simulink model "fxpdemo_sfun_user_U32BitRegion"  (Simulink 7.6)
settings: Solver=FixedStepDiscrete  StartTime=0.0  StopTime=1  FixedStep=0.001  RelTol=1e-3
libraries: simulink x8
settings Model: Creator=The MathWorks Inc.  ExtModeAutoUpdateStatusClock=off
settings OptimizationCC: InitFltsAndDblsToZero=on
settings DebuggingCC: StrictBusMsg=Warning

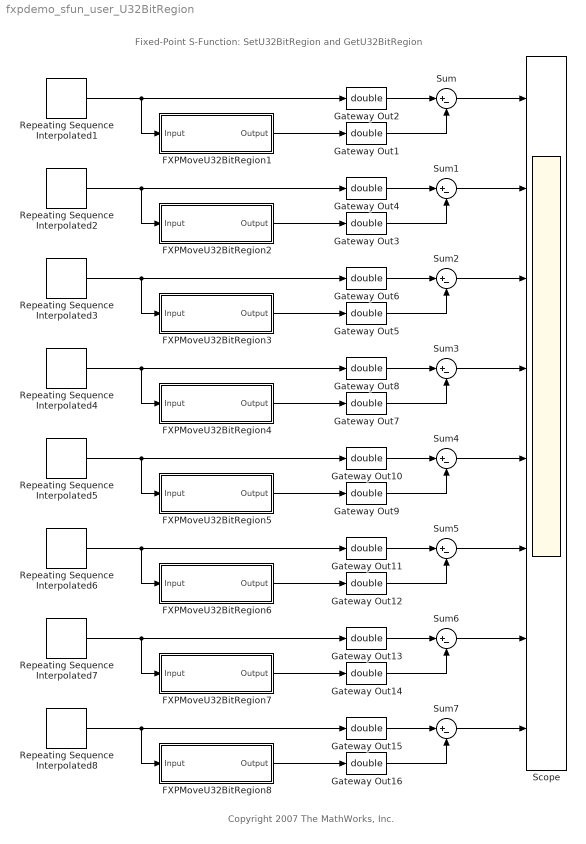
== system fxpdemo_sfun_user_U32BitRegion ==
  note: Fixed-Point S-Function: SetU32BitRegion and GetU32BitRegion
  note: Copyright 2007 The MathWorks, Inc.
  FXPMoveU32BitRegion1 : Subsystem
  FXPMoveU32BitRegion2 : Subsystem
  FXPMoveU32BitRegion3 : Subsystem
  FXPMoveU32BitRegion4 : Subsystem
  FXPMoveU32BitRegion5 : Subsystem
  FXPMoveU32BitRegion6 : Subsystem
  FXPMoveU32BitRegion7 : Subsystem
  FXPMoveU32BitRegion8 : Subsystem
  Gateway Out{1..16} (16 alike) : DataTypeConversion  OutDataTypeStr=double  RndMeth=Zero
  Repeating Sequence Interpolated1 : simulink/Sources/Repeating Sequence Interpolated  SystemSampleTime=-1  OutValues=0+2*[0 0.25 0.5 0.75 1].'  TimeValues=[0 0.25 0.5 0.75 1].'  LookUpMeth=Interpolation-Use End Values  tsamp=0.001  OutMin=[]  OutMax=[]  OutDataTypeStr=fixdt(0,9,4)  OutputDataTypeScalingMode=Specify via dialog  OutDataType=ufix(9)  OutScaling=2^-4
  Repeating Sequence Interpolated2 : simulink/Sources/Repeating Sequence Interpolated  SystemSampleTime=-1  OutValues=0+2*[0 0.25 0.5 0.75 1].'  TimeValues=[0 0.25 0.5 0.75 1].'  LookUpMeth=Interpolation-Use End Values  tsamp=0.001  OutMin=[]  OutMax=[]  OutDataTypeStr=fixdt(0,17,6)  OutputDataTypeScalingMode=Specify via dialog  OutDataType=ufix(17)  OutScaling=2^-6
  Repeating Sequence Interpolated3 : simulink/Sources/Repeating Sequence Interpolated  SystemSampleTime=-1  OutValues=0+2*[0 0.25 0.5 0.75 1].'  TimeValues=[0 0.25 0.5 0.75 1].'  LookUpMeth=Interpolation-Use End Values  tsamp=0.001  OutMin=[]  OutMax=[]  OutDataTypeStr=fixdt(0,33,8)  OutputDataTypeScalingMode=Specify via dialog  OutDataType=ufix(33)  OutScaling=2^-8
  Repeating Sequence Interpolated4 : simulink/Sources/Repeating Sequence Interpolated  SystemSampleTime=-1  OutValues=0+2*[0 0.25 0.5 0.75 1].'  TimeValues=[0 0.25 0.5 0.75 1].'  LookUpMeth=Interpolation-Use End Values  tsamp=0.001  OutMin=[]  OutMax=[]  OutDataTypeStr=fixdt(0,65,10)  OutputDataTypeScalingMode=Specify via dialog  OutDataType=ufix(65)  OutScaling=2^-10
  Repeating Sequence Interpolated5 : simulink/Sources/Repeating Sequence Interpolated  SystemSampleTime=-1  OutValues=0+2*[0 0.25 0.5 0.75 1].'  TimeValues=[0 0.25 0.5 0.75 1].'  LookUpMeth=Interpolation-Use End Values  tsamp=0.001  OutMin=[]  OutMax=[]  OutDataTypeStr=fixdt(1,15,3)  OutputDataTypeScalingMode=Specify via dialog  OutDataType=sfix(15)  OutScaling=2^-3
  Repeating Sequence Interpolated6 : simulink/Sources/Repeating Sequence Interpolated  SystemSampleTime=-1  OutValues=0+2*[0 0.25 0.5 0.75 1].'  TimeValues=[0 0.25 0.5 0.75 1].'  LookUpMeth=Interpolation-Use End Values  tsamp=0.001  OutMin=[]  OutMax=[]  OutDataTypeStr=fixdt(1,31,6)  OutputDataTypeScalingMode=Specify via dialog  OutDataType=sfix(31)  OutScaling=2^-6
  Repeating Sequence Interpolated7 : simulink/Sources/Repeating Sequence Interpolated  SystemSampleTime=-1  OutValues=0+2*[0 0.25 0.5 0.75 1].'  TimeValues=[0 0.25 0.5 0.75 1].'  LookUpMeth=Interpolation-Use End Values  tsamp=0.001  OutMin=[]  OutMax=[]  OutDataTypeStr=fixdt(1,63,9)  OutputDataTypeScalingMode=Specify via dialog  OutDataType=sfix(63)  OutScaling=2^-9
  Repeating Sequence Interpolated8 : simulink/Sources/Repeating Sequence Interpolated  SystemSampleTime=-1  OutValues=0+2*[0 0.25 0.5 0.75 1].'  TimeValues=[0 0.25 0.5 0.75 1].'  LookUpMeth=Interpolation-Use End Values  tsamp=0.001  OutMin=[]  OutMax=[]  OutDataTypeStr=fixdt(1,127,12)  OutputDataTypeScalingMode=Specify via dialog  OutDataType=sfix(127)  OutScaling=2^-12
  Scope : Scope  NumInputPorts=8
      settings: YMin=-5~-5~-5~-5~-5~-5~-5~-5  YMax=5~5~5~5~5~5~5~5
  Sum{,1..7} (8 alike) : Sum  Inputs=|+-
  wires:
  Repeating Sequence Interpolated1/1 -> Gateway Out2/1, FXPMoveU32BitRegion1/1(Input)
  FXPMoveU32BitRegion1/1(Output) -> Gateway Out1/1
  Gateway Out2/1 -> Sum/1
  Gateway Out1/1 -> Sum/2
  Repeating Sequence Interpolated2/1 -> FXPMoveU32BitRegion2/1(Input), Gateway Out4/1
  FXPMoveU32BitRegion2/1(Output) -> Gateway Out3/1
  Gateway Out4/1 -> Sum1/1
  Gateway Out3/1 -> Sum1/2
  Repeating Sequence Interpolated3/1 -> Gateway Out6/1, FXPMoveU32BitRegion3/1(Input)
  FXPMoveU32BitRegion3/1(Output) -> Gateway Out5/1
  Gateway Out6/1 -> Sum2/1
  Gateway Out5/1 -> Sum2/2
  Repeating Sequence Interpolated4/1 -> FXPMoveU32BitRegion4/1(Input), Gateway Out8/1
  FXPMoveU32BitRegion4/1(Output) -> Gateway Out7/1
  Gateway Out8/1 -> Sum3/1
  Gateway Out7/1 -> Sum3/2
  Repeating Sequence Interpolated5/1 -> Gateway Out10/1, FXPMoveU32BitRegion5/1(Input)
  FXPMoveU32BitRegion5/1(Output) -> Gateway Out9/1
  Gateway Out10/1 -> Sum4/1
  Gateway Out9/1 -> Sum4/2
  Repeating Sequence Interpolated6/1 -> FXPMoveU32BitRegion6/1(Input), Gateway Out11/1
  FXPMoveU32BitRegion6/1(Output) -> Gateway Out12/1
  Gateway Out11/1 -> Sum5/1
  Gateway Out12/1 -> Sum5/2
  Repeating Sequence Interpolated7/1 -> Gateway Out13/1, FXPMoveU32BitRegion7/1(Input)
  FXPMoveU32BitRegion7/1(Output) -> Gateway Out14/1
  Gateway Out13/1 -> Sum6/1
  Gateway Out14/1 -> Sum6/2
  Repeating Sequence Interpolated8/1 -> FXPMoveU32BitRegion8/1(Input), Gateway Out15/1
  FXPMoveU32BitRegion8/1(Output) -> Gateway Out16/1
  Gateway Out15/1 -> Sum7/1
  Gateway Out16/1 -> Sum7/2
  Sum/1 -> Scope/1
  Sum1/1 -> Scope/2
  Sum2/1 -> Scope/3
  Sum3/1 -> Scope/4
  Sum4/1 -> Scope/5
  Sum5/1 -> Scope/6
  Sum6/1 -> Scope/7
  Sum7/1 -> Scope/8

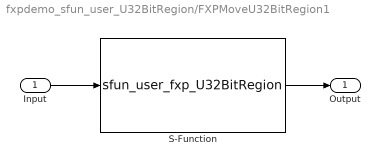
== system fxpdemo_sfun_user_U32BitRegion/FXPMoveU32BitRegion1 ==
  Input : Inport
  S-Function : S-Function  FunctionName=sfun_user_fxp_U32BitRegion  EnableBusSupport=off
  Output : Outport
  wires:
  Input/1 -> S-Function/1
  S-Function/1 -> Output/1

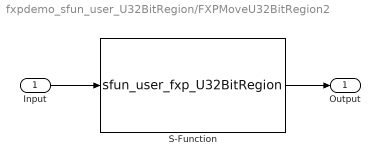
== system fxpdemo_sfun_user_U32BitRegion/FXPMoveU32BitRegion2 ==
  Input : Inport
  S-Function : S-Function  FunctionName=sfun_user_fxp_U32BitRegion  EnableBusSupport=off
  Output : Outport
  wires:
  S-Function/1 -> Output/1
  Input/1 -> S-Function/1

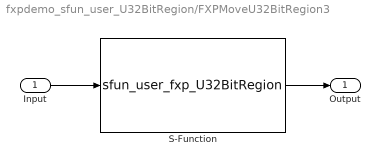
== system fxpdemo_sfun_user_U32BitRegion/FXPMoveU32BitRegion3 ==
  Input : Inport
  S-Function : S-Function  FunctionName=sfun_user_fxp_U32BitRegion  EnableBusSupport=off
  Output : Outport
  wires:
  Input/1 -> S-Function/1
  S-Function/1 -> Output/1

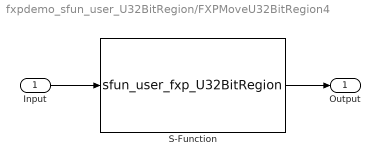
== system fxpdemo_sfun_user_U32BitRegion/FXPMoveU32BitRegion4 ==
  Input : Inport
  S-Function : S-Function  FunctionName=sfun_user_fxp_U32BitRegion  EnableBusSupport=off
  Output : Outport
  wires:
  S-Function/1 -> Output/1
  Input/1 -> S-Function/1

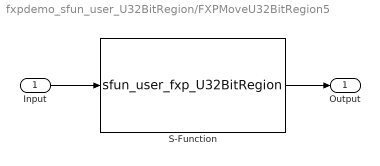
== system fxpdemo_sfun_user_U32BitRegion/FXPMoveU32BitRegion5 ==
  Input : Inport
  S-Function : S-Function  FunctionName=sfun_user_fxp_U32BitRegion  EnableBusSupport=off
  Output : Outport
  wires:
  Input/1 -> S-Function/1
  S-Function/1 -> Output/1

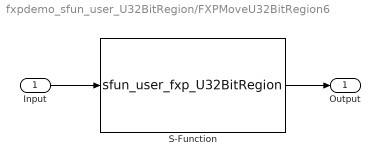
== system fxpdemo_sfun_user_U32BitRegion/FXPMoveU32BitRegion6 ==
  Input : Inport
  S-Function : S-Function  FunctionName=sfun_user_fxp_U32BitRegion  EnableBusSupport=off
  Output : Outport
  wires:
  S-Function/1 -> Output/1
  Input/1 -> S-Function/1

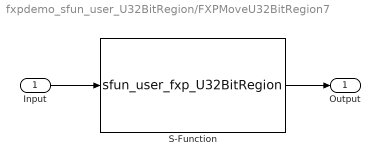
== system fxpdemo_sfun_user_U32BitRegion/FXPMoveU32BitRegion7 ==
  Input : Inport
  S-Function : S-Function  FunctionName=sfun_user_fxp_U32BitRegion  EnableBusSupport=off
  Output : Outport
  wires:
  Input/1 -> S-Function/1
  S-Function/1 -> Output/1

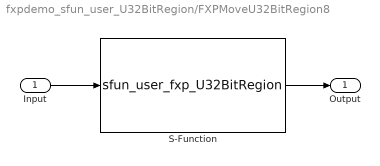
== system fxpdemo_sfun_user_U32BitRegion/FXPMoveU32BitRegion8 ==
  Input : Inport
  S-Function : S-Function  FunctionName=sfun_user_fxp_U32BitRegion  EnableBusSupport=off
  Output : Outport
  wires:
  S-Function/1 -> Output/1
  Input/1 -> S-Function/1
